simulink subsystem "PD_control"  (R2022b)
settings: Solver=VariableStepAuto  StartTime=0.0  StopTime=10.0  RelTol=1e-3
model mask{P=200, D=-0.1, G=-13}
  mask prompts: P "比例系数"; D "阻尼系数"; G "重力补偿"
settings Model: Creator=Administrator  LastModifiedBy=LiAn

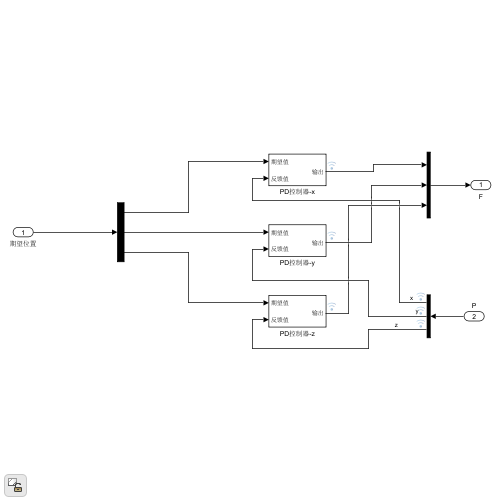
[thumbnail: Simulink's stored preview of the top-level diagram]
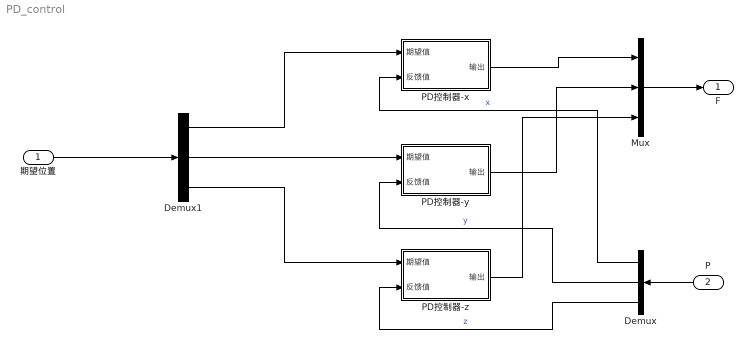
== system PD_control ==
  期望位置 : Inport
  P : Inport  Port=2
  Demux : Demux  Outputs=3
  Demux1 : Demux  Outputs=3
  Mux : Mux  Inputs=3
  PD控制器-x : Subsystem
  PD控制器-y : Subsystem
  PD控制器-z : Subsystem
  F : Outport
  wires:
  PD控制器-z/1(输出) -> Mux/3
  Mux/1 -> F/1
  Demux1/2 -> PD控制器-y/1(期望值)
  PD控制器-y/1(输出) -> Mux/2
  P/1 -> Demux/1
  Demux1/3 -> PD控制器-z/1(期望值)
  Demux1/1 -> PD控制器-x/1(期望值)
  Demux/1 -> PD控制器-x/2(反馈值)  "x"
  Demux/3 -> PD控制器-z/2(反馈值)  "z"
  Demux/2 -> PD控制器-y/2(反馈值)  "y"
  PD控制器-x/1(输出) -> Mux/1
  期望位置/1 -> Demux1/1

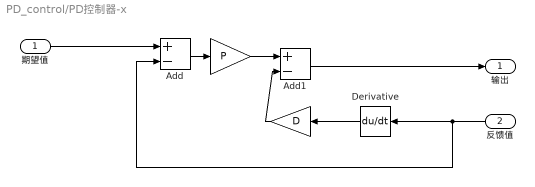
== system PD_control/PD控制器-x ==
  期望值 : Inport
  反馈值 : Inport  Port=2
  " " : Gain  Gain=P
  "    " : Gain  Gain=D
  Add : Sum  Inputs=+-
  Add1 : Sum  Inputs=+-
  Derivative : Derivative
  输出 : Outport
  wires:
  " "/1 -> Add1/1
  期望值/1 -> Add/1
  "    "/1 -> Add1/2
  Derivative/1 -> "    "/1
  Add/1 -> " "/1
  Add1/1 -> 输出/1
  反馈值/1 -> Add/2, Derivative/1

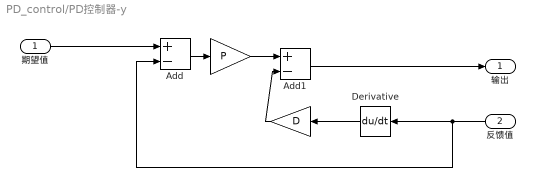
== system PD_control/PD控制器-y ==
  期望值 : Inport
  反馈值 : Inport  Port=2
  " " : Gain  Gain=P
  "    " : Gain  Gain=D
  Add : Sum  Inputs=+-
  Add1 : Sum  Inputs=+-
  Derivative : Derivative
  输出 : Outport
  wires:
  反馈值/1 -> Derivative/1, Add/2
  Add1/1 -> 输出/1
  Add/1 -> " "/1
  Derivative/1 -> "    "/1
  "    "/1 -> Add1/2
  期望值/1 -> Add/1
  " "/1 -> Add1/1

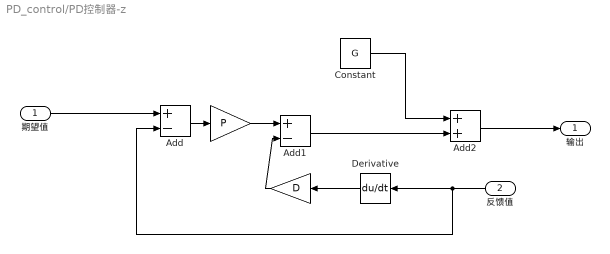
== system PD_control/PD控制器-z ==
  期望值 : Inport
  反馈值 : Inport  Port=2
  " " : Gain  Gain=P
  "    " : Gain  Gain=D
  Add : Sum  Inputs=+-
  Add1 : Sum  Inputs=+-
  Add2 : Sum
  Constant : Constant  Value=G
  Derivative : Derivative
  输出 : Outport
  wires:
  Constant/1 -> Add2/1
  Add2/1 -> 输出/1
  Add1/1 -> Add2/2
  " "/1 -> Add1/1
  期望值/1 -> Add/1
  "    "/1 -> Add1/2
  Derivative/1 -> "    "/1
  Add/1 -> " "/1
  反馈值/1 -> Add/2, Derivative/1
